simulink model "Project"  (R2023b)
settings: Solver=FixedStepAuto  StartTime=0.0  StopTime=5  FixedStep=1e-2  RelTol=1e-3
InitFcn:
  | Mmin = 0.5;
  | Mmax = 2;
  | Bmin = 0.2;
  | Bmax = 2;
  | Taumin = 0.001;
  | Taumax = 0.002;
undefined symbols (not defined in the file): peopleSoftNumber
libraries: simulink x1, uavutilslib x1
settings Model: Creator=arnoldpretorius  LastModifiedBy=arnoldpretorius
settings OptimizationCC: ReuseModelBlockBuffer=off
settings DebuggingCC: UnconnectedInputMsg=warning  UnconnectedOutputMsg=warning  UnconnectedLineMsg=warning
settings ModelReferenceCC: EnableRefExpFcnMdlSchedulingChecks=on
settings RTWCC: DLArmComputeVersion=19.05

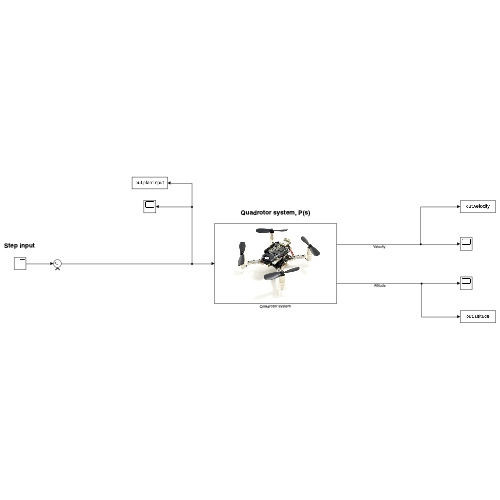
[thumbnail: Simulink's stored preview of the top-level diagram]
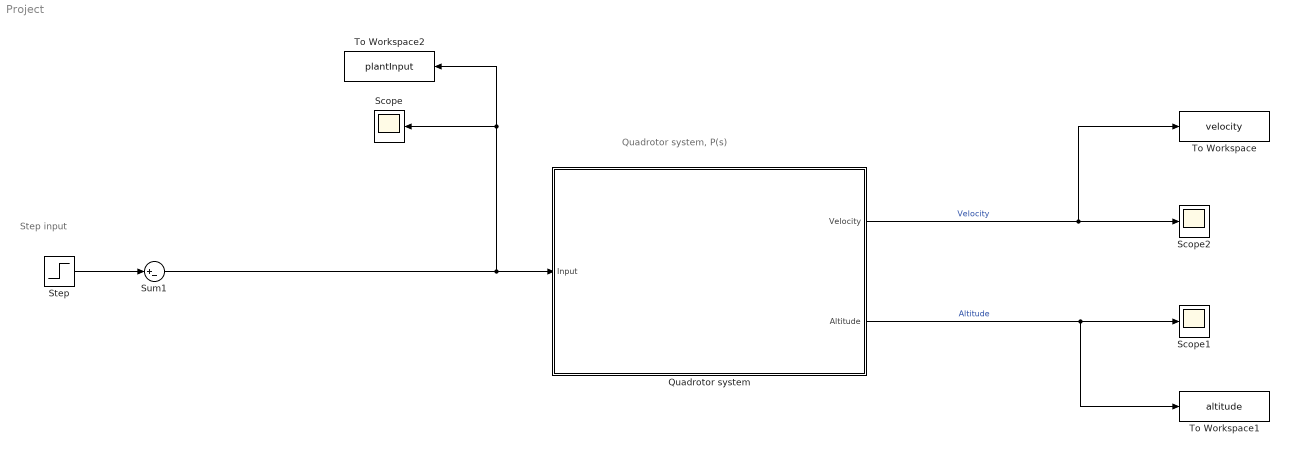
== system Project ==
  note: Step input
  note: Quadrotor system, P(s)
  Quadrotor system : Subsystem
      mask Display: image('$imagefile'); % Use "Edit Image" on toolstrip to change.
  Scope : Scope
  Scope1 : Scope
  Scope2 : Scope
  Step : Step  Time=0  After=0  SampleTime=0
  Sum1 : Sum  Inputs=|+-
  To Workspace : ToWorkspace  VariableName=velocity  SaveFormat=Timeseries  SampleTime=-1
  To Workspace1 : ToWorkspace  VariableName=altitude  SaveFormat=Timeseries  SampleTime=-1
  To Workspace2 : ToWorkspace  VariableName=plantInput  SaveFormat=Timeseries  SampleTime=-1
  wires:
  Quadrotor system/1(Velocity) -> Scope2/1, To Workspace/1  "Velocity"
  Quadrotor system/2(Altitude) -> Scope1/1, To Workspace1/1  "Altitude"
  Step/1 -> Sum1/1
  Sum1/1 -> Scope/1, To Workspace2/1, Quadrotor system/1(Input)

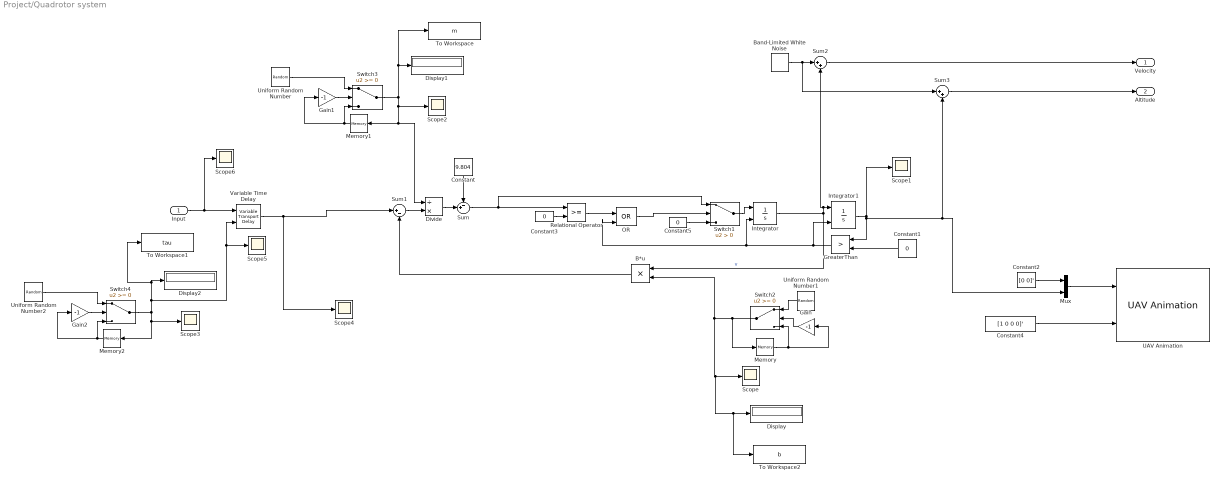
== system Project/Quadrotor system ==
  Input : Inport
  B*u : Product  Inputs=**
  Band-Limited White Noise : simulink/Sources/Band-Limited White Noise  Cov=[0.0001]  Ts=0.1  seed=[23341]
  Constant : Constant  Value=9.804
  Constant1 : Constant  Value=0
  Constant2 : Constant  Value=[0 0]'
  Constant3 : Constant  Value=0
  Constant4 : Constant  Value=[1 0 0 0]'
  Constant5 : Constant  Value=0
  Display : Display
  Display1 : Display
  Display2 : Display
  Divide : Product  Inputs=/*
  Gain : Gain  Gain=-1
  Gain1 : Gain  Gain=-1
  Gain2 : Gain  Gain=-1
  GreaterThan : RelationalOperator  Operator=>  OutDataTypeStr=boolean  RndMeth=Simplest  InputSameDT=off
  Integrator : Integrator  ExternalReset=falling  ContinuousStateAttributes='velocity'
  Integrator1 : Integrator  ExternalReset=falling
  Memory : Memory
  Memory1 : Memory
  Memory2 : Memory
  Mux : Mux  Inputs=2
  OR : Logic  Operator=OR  IconShape=distinctive  AllPortsSameDT=off  OutDataTypeStr=boolean
  Relational Operator : RelationalOperator  OutDataTypeStr=boolean  RndMeth=Simplest  InputSameDT=off
  Scope{,1..6} (7 alike) : Scope
  Sum : Sum  Inputs=-+|
  Sum1 : Sum  Inputs=|+-
  Sum2 : Sum  Inputs=|++
  Sum3 : Sum  Inputs=|++
  Switch1 : Switch  Criteria=u2 > Threshold  SaturateOnIntegerOverflow=off  InputSameDT=off
  Switch2 : Switch  SaturateOnIntegerOverflow=off  InputSameDT=off
  Switch3 : Switch  SaturateOnIntegerOverflow=off  InputSameDT=off
  Switch4 : Switch  SaturateOnIntegerOverflow=off  InputSameDT=off
  To Workspace : ToWorkspace  VariableName=m  SaveFormat=Timeseries  SampleTime=-1
  To Workspace1 : ToWorkspace  VariableName=tau  SaveFormat=Timeseries  SampleTime=-1
  To Workspace2 : ToWorkspace  VariableName=b  SaveFormat=Timeseries  SampleTime=-1
  UAV Animation : uavutilslib/UAV Animation  UAVType=Multirotor  UAVSize=1  InertialZDirection=Up  SampleTime=-1
  Uniform Random Number : UniformRandomNumber  Minimum=Mmin  Maximum=Mmax  Seed=peopleSoftNumber  SampleTime=0.1
  Uniform Random Number1 : UniformRandomNumber  Minimum=Bmin  Maximum=Bmax  Seed=peopleSoftNumber+1  SampleTime=0.1
  Uniform Random Number2 : UniformRandomNumber  Minimum=Taumin  Maximum=Taumax  Seed=peopleSoftNumber  SampleTime=0.1
  Variable Time Delay : VariableTransportDelay  MaximumDelay=10
  Velocity : Outport
  Altitude : Outport  Port=2
  wires:
  Constant4/1 -> UAV Animation/2
  Sum1/1 -> Divide/2
  Mux/1 -> UAV Animation/1
  B*u/1 -> Sum1/2
  Integrator1/1 -> GreaterThan/1, Sum3/2, Mux/2, Scope1/1
  Constant2/1 -> Mux/1
  Constant1/1 -> GreaterThan/2
  Switch3/1 -> To Workspace/1, Display1/1, Scope2/1, Memory1/1, Divide/1
  Switch2/1 -> Memory/1, To Workspace2/1, Display/1, Scope/1, B*u/2
  Uniform Random Number1/1 -> Switch2/1
  Memory/1 -> Gain/1, Switch2/3
  Gain/1 -> Switch2/2
  Gain1/1 -> Switch3/2
  Uniform Random Number/1 -> Switch3/1
  Memory1/1 -> Gain1/1, Switch3/3
  Constant/1 -> Sum/1
  Divide/1 -> Sum/2
  GreaterThan/1 -> Integrator1/2, Integrator/2, OR/2
  Sum/1 -> Switch1/1, Relational Operator/1
  Relational Operator/1 -> OR/1
  Constant5/1 -> Switch1/3
  Integrator/1 -> Sum2/2, Integrator1/1, B*u/1  "v"
  Constant3/1 -> Relational Operator/2
  OR/1 -> Switch1/2
  Switch1/1 -> Integrator/1
  Band-Limited White Noise/1 -> Sum3/1, Sum2/1
  Sum2/1 -> Velocity/1
  Sum3/1 -> Altitude/1
  Uniform Random Number2/1 -> Switch4/1
  Gain2/1 -> Switch4/2
  Switch4/1 -> Scope5/1, Variable Time Delay/2, To Workspace1/1, Display2/1, Memory2/1, Scope3/1
  Memory2/1 -> Gain2/1, Switch4/3
  Input/1 -> Scope6/1, Variable Time Delay/1
  Variable Time Delay/1 -> Scope4/1, Sum1/1
